simulink model "task_01_3"  (R2021b)
settings: Solver=VariableStepAuto  StartTime=0.0  StopTime=10.0  RelTol=1e-3
settings Model: Creator=User_Admin  LastModifiedBy=User_Admin

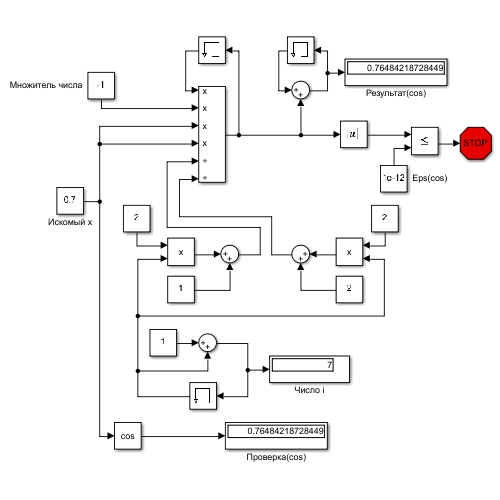
[thumbnail: Simulink's stored preview of the top-level diagram]
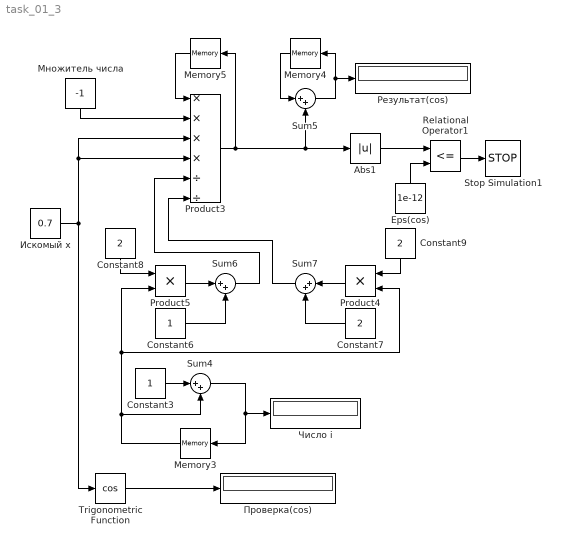
== system task_01_3 ==
  Abs1 : Abs
  Constant3 : Constant
  Constant6 : Constant
  Constant7 : Constant  Value=2
  Constant8 : Constant  Value=2
  Constant9 : Constant  Value=2
  Eps(cos) : Constant  Value=1e-12
  Memory3 : Memory
  Memory4 : Memory  InitialCondition=1
  Memory5 : Memory  InitialCondition=1
  Product3 : Product  Inputs=****//
  Product4 : Product
  Product5 : Product
  Relational Operator1 : RelationalOperator  Operator=<=  OutDataTypeStr=boolean  RndMeth=Simplest
  Stop Simulation1 : Stop
  Sum{4..7} (4 alike) : Sum  Inputs=|++
  Trigonometric Function : Trigonometry  Operator=cos
  Искомый х : Constant  Value=0.7
  Множитель числа : Constant  Value=-1
  Проверка(cos) : Display
  Результат(cos) : Display
  Число i : Display
  wires:
  Sum6/1 -> Product3/5
  Sum4/1 -> Memory3/1, Число i/1
  Constant3/1 -> Sum4/1
  Constant8/1 -> Product5/1
  Product5/1 -> Sum6/1
  Constant7/1 -> Sum7/2
  Sum5/1 -> Memory4/1, Результат(cos)/1
  Множитель числа/1 -> Product3/2
  Sum7/1 -> Product3/6
  Constant9/1 -> Product4/1
  Memory3/1 -> Sum4/2, Product5/2, Product4/2
  Искомый х/1 -> Trigonometric Function/1, Product3/3, Product3/4
  Eps(cos)/1 -> Relational Operator1/2
  Product3/1 -> Sum5/2, Abs1/1, Memory5/1
  Memory4/1 -> Sum5/1
  Memory5/1 -> Product3/1
  Relational Operator1/1 -> Stop Simulation1/1
  Product4/1 -> Sum7/1
  Trigonometric Function/1 -> Проверка(cos)/1
  Constant6/1 -> Sum6/2
  Abs1/1 -> Relational Operator1/1
